simulink model "simulinkmodel"  (R2021b)
settings: Solver=VariableStepAuto  StartTime=0.0  StopTime=100  RelTol=1e-3
libraries: fuzblock x1
settings Model: Creator=radov  LastModifiedBy=radov

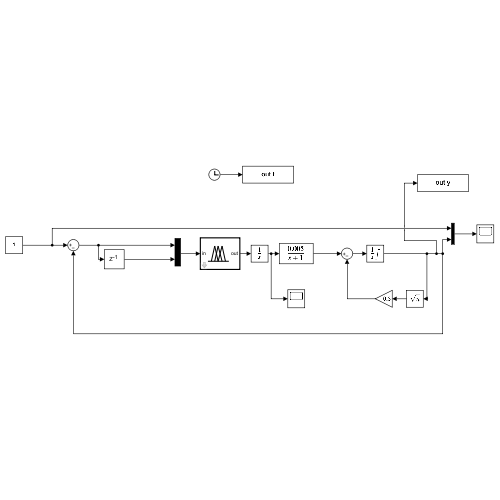
[thumbnail: Simulink's stored preview of the top-level diagram]
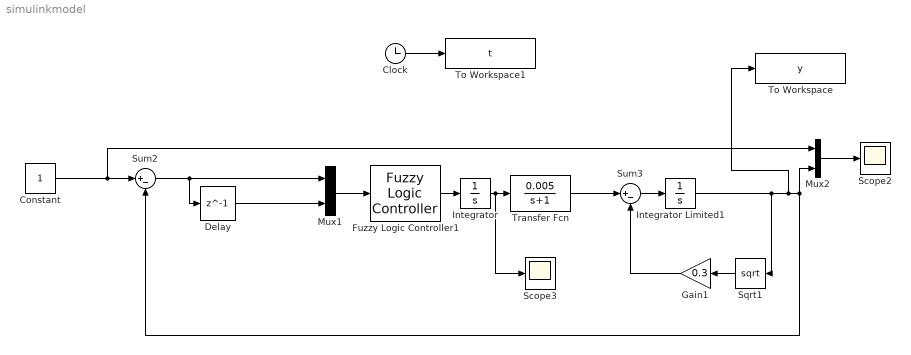
== system simulinkmodel ==
  Clock : Clock
  Constant : Constant
  Delay : Delay  DelayLength=1
  Fuzzy Logic Controller1 : fuzblock/Fuzzy Logic  Controller  FIS=valvePI  OutputSampleNumber=101  DataType=double  FuzzifiedInputs=off  RuleFiringStrengths=off  RuleOutputs=off  AggregatedOutputs=off  SimulateUsing=Interpreted execution  OutOfRangeInputValueMessage=warning  NoRuleFiredMessage=warning  EmptyOutputFuzzySetMessage=warning
  Gain1 : Gain  Gain=0.3
  Integrator : Integrator
  Integrator Limited1 : Integrator  LimitOutput=on  UpperSaturationLimit=1  LowerSaturationLimit=-1
  Mux1 : Mux  Inputs=2
  Mux2 : Mux  Inputs=2
  Scope2 : Scope
  Scope3 : Scope
  Sqrt1 : Sqrt  SaturateOnIntegerOverflow=on
  Sum2 : Sum  Inputs=|+-
  Sum3 : Sum  Inputs=|+-
  To Workspace : ToWorkspace  VariableName=y  SaveFormat=Timeseries  SampleTime=-1
  To Workspace1 : ToWorkspace  VariableName=t  SaveFormat=Timeseries
  Transfer Fcn : TransferFcn  Numerator=[0.005]  Denominator=[1 1]
  wires:
  Constant/1 -> Mux2/1, Sum2/1
  Transfer Fcn/1 -> Sum3/1
  Sum3/1 -> Integrator Limited1/1
  Sqrt1/1 -> Gain1/1
  Integrator Limited1/1 -> To Workspace/1, Mux2/2, Sum2/2, Sqrt1/1
  Gain1/1 -> Sum3/2
  Mux2/1 -> Scope2/1
  Mux1/1 -> Fuzzy Logic Controller1/1
  Sum2/1 -> Delay/1, Mux1/1
  Delay/1 -> Mux1/2
  Fuzzy Logic Controller1/1 -> Integrator/1
  Integrator/1 -> Transfer Fcn/1, Scope3/1
  Clock/1 -> To Workspace1/1
